simulink model "sixdof_vel"  (R2020b)
settings: Solver=FixedStepAuto  StartTime=0.0  StopTime=20  FixedStep=0.00001  RelTol=1e-3
libraries: shared6dof x1
settings Model: Creator=rajat  LastModifiedBy=rajat

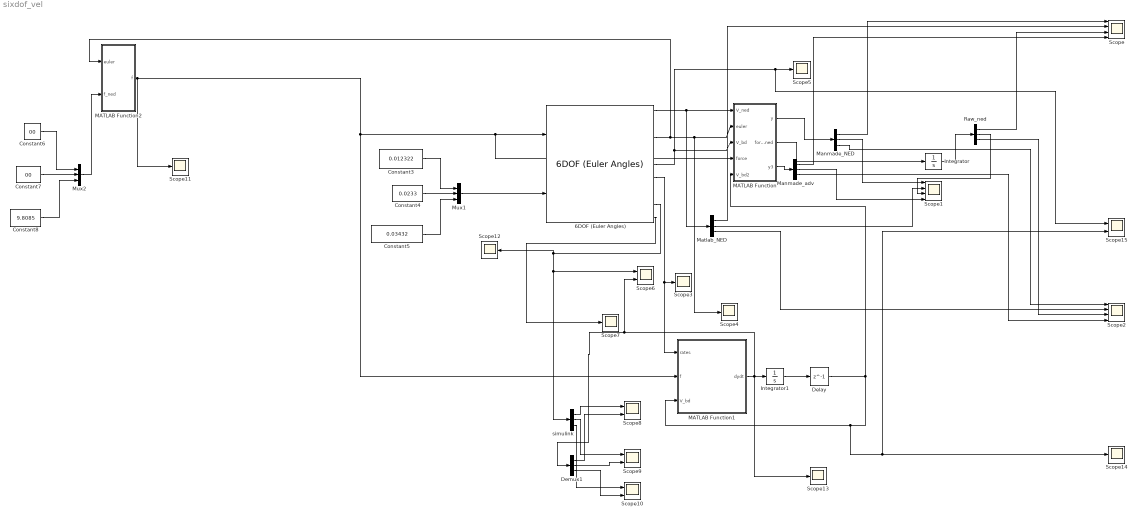
== system sixdof_vel ==
  6DOF (Euler Angles) : shared6dof/6DOF (Euler Angles)  units=Metric (MKS)  mtype=Fixed  rep=Euler Angles  xme_0=[0 0 0]  Vm_0=[0 0 0]  eul_0=[0 0 0]  pm_0=[0 0 0]  mass_0=1.0  mass_e=0.5  mass_f=2.0  inertia=eye(3)  inertia_e=eye(3)  inertia_f=2*eye(3)  k_quat=1.0  vre_flag=on  abi_flag=on  aMode=0  xme_statename=''  Vm_statename=''  eul_statename=''  quat_statename=''  pm_statename=''  mass_statename=''
      settings: SourceProductBaseCode=AE,PW,MT,UV,VE,VP
  Constant3 : Constant  Value=0.012322
  Constant4 : Constant  Value=0.0233
  Constant5 : Constant  Value=0.03432
  Constant6 : Constant  Value=00
  Constant7 : Constant  Value=00
  Constant8 : Constant  Value=9.8085
  Delay : Delay  DelayLength=1
  Demux1 : Demux  Outputs=3
  Integrator : Integrator
  Integrator1 : Integrator
  MATLAB Function : MATLAB Function  TreatAsAtomicUnit=on
  MATLAB Function1 : MATLAB Function  TreatAsAtomicUnit=on
  MATLAB Function2 : MATLAB Function  TreatAsAtomicUnit=on
  Manmade_NED : Demux  Outputs=3
  Manmade_adv : Demux  Outputs=3
  Matlab_NED : Demux  Outputs=3
  Mux1 : Mux  Inputs=3
  Mux2 : Mux  Inputs=3
  Raw_ned : Demux  Outputs=3
  Scope : Scope  NumInputPorts=4
  Scope1 : Scope  NumInputPorts=4
  Scope{6,8..10,15} (5 alike) : Scope  NumInputPorts=2
  Scope{3..5,7,11..14} (8 alike) : Scope
  Scope2 : Scope  NumInputPorts=4
  simulink : Demux  Outputs=3
  wires:
  Mux1/1 -> 6DOF (Euler Angles)/2
  Constant5/1 -> Mux1/3
  Constant3/1 -> Mux1/1
  Constant4/1 -> Mux1/2
  6DOF (Euler Angles)/1 -> Matlab_NED/1, MATLAB Function/1(V_ned)
  MATLAB Function/1(y) -> Manmade_NED/1
  Manmade_NED/1 -> Scope/1
  Matlab_NED/1 -> Scope/2
  Manmade_NED/2 -> Scope1/1
  Matlab_NED/2 -> Scope1/2
  Manmade_NED/3 -> Scope2/1
  Matlab_NED/3 -> Scope2/2
  6DOF (Euler Angles)/3 -> MATLAB Function2/1(euler), Scope4/1, MATLAB Function/2(euler)
  6DOF (Euler Angles)/5 -> Scope15/1, Scope5/1, MATLAB Function/3(V_bd)
  6DOF (Euler Angles)/6 -> MATLAB Function1/1(rates), Scope3/1
  MATLAB Function/2(force_ned) -> Integrator/1
  Integrator/1 -> Raw_ned/1
  Raw_ned/1 -> Scope/3
  Raw_ned/2 -> Scope1/3
  Raw_ned/3 -> Scope2/3
  MATLAB Function1/1(dydt) -> Scope13/1, Demux1/1, Scope6/2, Integrator1/1
  Integrator1/1 -> Delay/1
  Delay/1 -> MATLAB Function/5(V_bd2), Scope15/2, Scope14/1, MATLAB Function1/3(V_bd)
  MATLAB Function/3(y3) -> Manmade_adv/1
  Manmade_adv/1 -> Scope/4
  Manmade_adv/2 -> Scope1/4
  Manmade_adv/3 -> Scope2/4
  6DOF (Euler Angles)/8 -> Scope6/1, simulink/1, Scope12/1
  6DOF (Euler Angles)/9 -> Scope7/1
  simulink/1 -> Scope8/1
  Demux1/1 -> Scope8/2
  simulink/2 -> Scope9/1
  Demux1/2 -> Scope9/2
  simulink/3 -> Scope10/1
  Demux1/3 -> Scope10/2
  MATLAB Function2/1(f) -> MATLAB Function1/2(f), MATLAB Function/4(force), 6DOF (Euler Angles)/1, Scope11/1
  Constant8/1 -> Mux2/3
  Constant6/1 -> Mux2/1
  Constant7/1 -> Mux2/2
  Mux2/1 -> MATLAB Function2/2(f_ned)

== matlab function sixdof_vel/MATLAB Function1 ==
  data: rates input; dydt output; f input; V_bd input
function dydt = fcn(rates, f, V_bd)

dydt=zeros(3,1);
mass_inv=1;
p=rates(1);
q=rates(2);
r=rates(3);
u=V_bd(1);
v=V_bd(2);
w=V_bd(3);



	dydt(1) = ((f(1)*mass_inv) + (r*v) - (q*w));%//%u_dot//optimization
	dydt(2) = ((f(2)*mass_inv) + (p*w) - (r*u));%//%v_dot
	dydt(3) = (f(3)*mass_inv) + (q*u) - (p*v);%//%w_dot

%dydt=zeros(3,1);
end

== matlab function sixdof_vel/MATLAB Function ==
  data: V_ned input; euler input; V_bd input; y output; force input; force_ned output; V_bd2 input; y3 output
function [y,force_ned,y3] = fcn(V_ned, euler, V_bd, force, V_bd2)

phi=euler(1);
theta=euler(2);
psi=euler(3);

R_v1_v= [  cos(psi),  sin(psi),  0 ;  ...
          -sin(psi),  cos(psi),  0;   ...
                 0 ,      0   ,  1  ] ;

 
R_v2_v1= [  cos(theta),   0,    -sin(theta); ...
                    0,    1,      0 ;        ...
           sin(theta),    0,     cos(theta)  ];
 
 
 
R_b_v2= [   1,     0,            0 ;        ...
           0,     cos(phi),     sin(phi) ; ...        
           0,    -sin(phi),     cos(phi)    ];
       
       
       
      y = (R_b_v2*R_v2_v1*R_v1_v)'*V_bd;
       
             y3 = (R_b_v2*R_v2_v1*R_v1_v)'*V_bd2;

       force_ned=(R_b_v2*R_v2_v1*R_v1_v)'*force;


end

== matlab function sixdof_vel/MATLAB Function2 ==
  data: euler input; f output; f_ned input
function f = fcn(euler,f_ned)

phi=euler(1);
theta=euler(2);
psi=euler(3);

R_v1_v= [  cos(psi),  sin(psi),  0 ;  ...
          -sin(psi),  cos(psi),  0;   ...
                 0 ,      0   ,  1  ] ;

 
R_v2_v1= [  cos(theta),   0,    -sin(theta); ...
                    0,    1,      0 ;        ...
           sin(theta),    0,     cos(theta)  ];
 
 
 
R_b_v2= [   1,     0,            0 ;        ...
           0,     cos(phi),     sin(phi) ; ...        
           0,    -sin(phi),     cos(phi)    ];
       
       
       
      f = (R_b_v2*R_v2_v1*R_v1_v)*f_ned;
      
      
end
